simulink model "TWIN"  (R2022a)
settings: Solver=FixedStepAuto  StartTime=0.0  StopTime=20  FixedStep=Ts  RelTol=1000000
values from neighbouring files (symbols this model uses):
  axis_A_init = X(1)    [MOSC_two_axis_machine_key.m]
  axis_B_init = Y(1)    [MOSC_two_axis_machine_key.m]
  c = 0    [MOSC_two_axis_machine_key.m]
  i_offset = 0.01    [MOSC_two_axis_machine_key.m]
  In = 7.2    [MOSC_two_axis_machine_key.m]
  J = (0.013*2)    (= 0.026)    [MOSC_two_axis_machine_key.m]
  k1a = 2    [MOSC_two_axis_machine_key.m]
  k1b = 2    [MOSC_two_axis_machine_key.m]
  k2a = 2    [MOSC_two_axis_machine_key.m]
  k2b = 2    [MOSC_two_axis_machine_key.m]
  k3b = 2    [MOSC_two_axis_machine_key.m]
  k4b = 2    [MOSC_two_axis_machine_key.m]
  k_conv = 350    [MOSC_two_axis_machine_key.m]
  k_meas_i = 10    [MOSC_two_axis_machine_key.m]
  k_meas_w = 5    [MOSC_two_axis_machine_key.m]
  Ki = Kr    (= 0.448835548336)    [MOSC_two_axis_machine_key.m]
  ki_om = K_reg_omega_SO    (= 0.938140461276)    [MOSC_two_axis_machine_key.m]
  Kp = Kr*Tr    (= 0.00161048636688)    [MOSC_two_axis_machine_key.m]
  kp_om = K_reg_omega_SO * T_reg_omega_SO    (= 0.185714285714)    [MOSC_two_axis_machine_key.m]
  kp_pos = 13    [MOSC_two_axis_machine_key.m]
  La = 23e-3    (= 0.023)    [MOSC_two_axis_machine_key.m]
  PSI_E = (Un-Ra*In)/wn    (= 1.36163652923)    [MOSC_two_axis_machine_key.m]
  PSI_M = Tn/In    (= 1.22916666667)    [MOSC_two_axis_machine_key.m]
  Ra = 6.41    [MOSC_two_axis_machine_key.m]
  rand_seed_1 = round(rand*(2^32-1))    [MOSC_two_axis_machine_key.m]
  rand_seed_2 = round(rand*(2^32-1))    [MOSC_two_axis_machine_key.m]
  rand_seed_3 = round(rand*(2^32-1))    [MOSC_two_axis_machine_key.m]
  rand_seed_4 = round(rand*(2^32-1))    [MOSC_two_axis_machine_key.m]
  Tdelay = 2*Ts    (= 0.002)    [MOSC_two_axis_machine_key.m]
  Tn = 8.85    [MOSC_two_axis_machine_key.m]
  Ts = 0.001    [MOSC_two_axis_machine_key.m]
  v_i_a = (In*measurement_noise_level/2)^2    (= 0.001296)    [MOSC_two_axis_machine_key.m]
  w1a = 1*2*pi*frequency_heart    (= 6.28318530718)    [MOSC_two_axis_machine_key.m]
  w1b = 1*2*pi*frequency_heart    (= 6.28318530718)    [MOSC_two_axis_machine_key.m]    (also in MOSC_updates.m = k(1)*1*2*pi*frequency_heart)
  w2a = 3*2*pi*frequency_heart    (= 18.8495559215)    [MOSC_two_axis_machine_key.m]
  w2b = 2*2*pi*frequency_heart    (= 12.5663706144)    [MOSC_two_axis_machine_key.m]    (also in MOSC_updates.m = k(2)*2*2*pi*frequency_heart)
  w3b = 3*2*pi*frequency_heart    (= 18.8495559215)    [MOSC_two_axis_machine_key.m]    (also in MOSC_updates.m = k(3)*3*2*pi*frequency_heart)
  w4b = 4*2*pi*frequency_heart    (= 25.1327412287)    [MOSC_two_axis_machine_key.m]    (also in MOSC_updates.m = k(4)*4*2*pi*frequency_heart)
  w_i_a = (dia_max*system_noise_level/2)^2    (= 2500)    [MOSC_two_axis_machine_key.m]
  w_offset = 0    [MOSC_two_axis_machine_key.m]
  w_omega_m = (domega_max*system_noise_level/2)^2    (= 100)    [MOSC_two_axis_machine_key.m]
  w_u_a = (du_max*system_noise_level/2)^2    (= 25000000)    [MOSC_two_axis_machine_key.m]
  wn = 1640*pi/30    (= 171.740398396)    [MOSC_two_axis_machine_key.m]
  zeta1a = 0.01    [MOSC_two_axis_machine_key.m]
  zeta1b = 0.01    [MOSC_two_axis_machine_key.m]
  zeta2a = 0.01    [MOSC_two_axis_machine_key.m]
  zeta2b = 0.01    [MOSC_two_axis_machine_key.m]
  zeta3b = 0.01    [MOSC_two_axis_machine_key.m]
  zeta4b = 0.01    [MOSC_two_axis_machine_key.m]
libraries: slpidlib x4
settings Model: Creator=nirvana1289  LastModifiedBy=akash
settings SolverCC: ZeroCrossAlgorithm=Adaptive  AlgebraicLoopSolver=TrustRegion
settings DataIOCC: ReturnWorkspaceOutputs=off
settings DebuggingCC: IgnoredZcDiagnostic=none  UnconnectedInputMsg=warning  UnconnectedOutputMsg=warning  UnconnectedLineMsg=warning  SFMachineParentedDataDiag=warning  ArithmeticOperatorsInVariantConditions=warning
settings SFSimCC: SimUseLocalCustomCode=off  CustomCodeUndefinedFunction=UseInterfaceOnly
settings RTWCC: RTWUseLocalCustomCode=off  DLArmComputeVersion=19.05
settings CodeAppCC: StateflowObjectComments=on

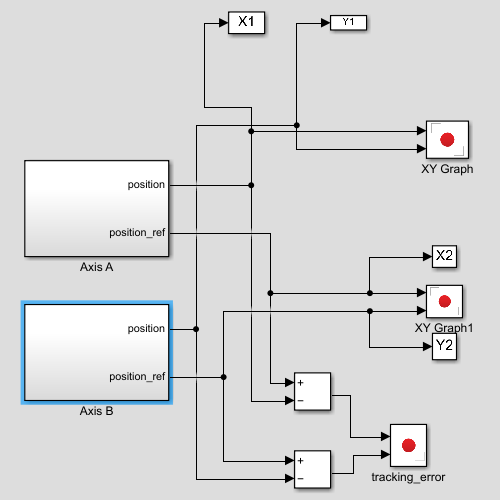
[thumbnail: Simulink's stored preview of the top-level diagram]
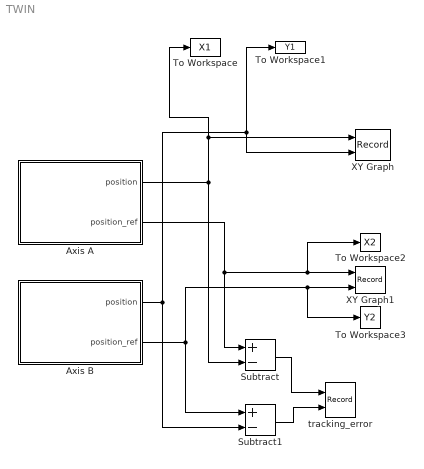
== system TWIN ==
  Axis A : Subsystem
  Axis B : Subsystem
  Subtract : Sum  Inputs=+-
  Subtract1 : Sum  Inputs=+-
  To Workspace : ToWorkspace  VariableName=X1  SampleTime=-1
      settings: Save2DSignal=2-D array (concatenate along first dimension)
  To Workspace1 : ToWorkspace  VariableName=Y1  SampleTime=-1
      settings: Save2DSignal=2-D array (concatenate along first dimension)
  To Workspace2 : ToWorkspace  VariableName=X2  SampleTime=-1
      settings: Save2DSignal=2-D array (concatenate along first dimension)
  To Workspace3 : ToWorkspace  VariableName=Y2  SampleTime=-1
      settings: Save2DSignal=2-D array (concatenate along first dimension)
  XY Graph : Record  FileSettingsInternal="{\"entries\":[{\"content\":{\"excelSettings\":{\"content\":{},\"type\":\"Streamout.ExcelSettings\"}},\"type\":\"Streamout.FileSettingStorage\",\"uuid\":\"5dd5c6a3-9558-46e3-9c57-18c47edfeb62\"}],\"packageUris\":[\"http://schema.mathworks.com/mf0/streamout_blocks/R2020a\"],\"version\":\"1.0\"}"  Layout=[1 1]  SignalsInternal="{\"entries\":[{\"content\":{\"signals\":[{\"content\":{\"blockPath\":[\"TWIN/XY Graph\"],\"channel\":[],\"dimensions\":[1],\"domain\":\"TWIN/XY Graph\",\"lineColor\":\"#a2142f\",\"plots\":[1],\"port\":1,\"sid\":[\"\"],\"signalID\":483759,\"signalName\":\"Axis A:1\"},\"type\":\"RecordBlkView.Signal\",\"uuid\":\"e5131e20-f6b1-48ad-bb87-b3fb0198be33\"},{\"content\":{\"blockPath\":[\"TWIN/XY Graph\"],\"channel\":[],\"dimensions\":[1],\"domain\":\"TWIN/XY Graph\",\"lineColor\":\"#139fff\",\"plots\":[1],\"port\":2,\"sid\":[\"\"],\"signalID\":483763,\"signalName\":\"Axis B:1\"},\"type\":\"RecordBlkView.Signal\",\"uuid\":\"a231155c-1ff8-46a4-b816-94ab751d59c2\"}]},\"type\":\"RecordBlkView.InputSignals\",\"uuid\":\"a1552bf6-88ac-4365-aa89-aa31ab89a906\"}],\"packageUris\":[\"http://schema.mathworks.com/mf0/streamout_blocks/R2020a\"],\"version\":\"1.0\"}"  VisualizationBindings="{\"xyplotplugin\":{\"info\":[{\"series\":[{\"bindingParametersList\":[{\"parameter\":\"X-Axis\",\"signalID\":483759,\"signalName\":\"Axis A:1\"},{\"parameter\":\"Y-Axis\",\"signalID\":483763,\"signalName\":\"Axis B:1\"}],\"seriesID\":45665}],\"subplotID\":1}]}}"  CompatibilityTag=XY
  XY Graph1 : Record  FileSettingsInternal="{\"entries\":[{\"content\":{\"excelSettings\":{\"content\":{},\"type\":\"Streamout.ExcelSettings\"}},\"type\":\"Streamout.FileSettingStorage\",\"uuid\":\"d2fb6019-1089-4865-91d9-d366b06b0246\"}],\"packageUris\":[\"http://schema.mathworks.com/mf0/streamout_blocks/R2020a\"],\"version\":\"1.0\"}"  Layout=[1 1]  SignalsInternal="{\"entries\":[{\"content\":{\"signals\":[{\"content\":{\"blockPath\":[\"TWIN/XY Graph1\"],\"channel\":[],\"dimensions\":[1],\"domain\":\"TWIN/XY Graph1\",\"lineColor\":\"#ff6929\",\"plots\":[],\"port\":1,\"sid\":[\"\"],\"signalID\":483767,\"signalName\":\"Axis A:2\"},\"type\":\"RecordBlkView.Signal\",\"uuid\":\"f7357322-d349-4bee-9fb2-232c0e5c727e\"},{\"content\":{\"blockPath\":[\"TWIN/XY Graph1\"],\"channel\":[],\"dimensions\":[1],\"domain\":\"TWIN/XY Graph1\",\"lineColor\":\"#b746ff\",\"plots\":[],\"port\":2,\"sid\":[\"\"],\"signalID\":483771,\"signalName\":\"Axis B:2\"},\"type\":\"RecordBlkView.Signal\",\"uuid\":\"1ed46889-5323-47ea-b6ba-a8126608ec68\"}]},\"type\":\"RecordBlkView.InputSignals\",\"uuid\":\"2741a743-7749-4c48-8803-007fd9de5a09\"}],\"packageUris\":[\"http://schema.mathworks.com/mf0/streamout_blocks/R2020a\"],\"version\":\"1.0\"}"  VisualizationBindings="{\"xyplotplugin\":{\"info\":[{\"series\":[],\"subplotID\":1}]}}"  CompatibilityTag=XY
  tracking_error : Record  FileSettingsInternal="{\"entries\":[{\"content\":{\"excelSettings\":{\"content\":{},\"type\":\"Streamout.ExcelSettings\"}},\"type\":\"Streamout.FileSettingStorage\",\"uuid\":\"68a8b464-3159-494c-9b13-e187b7557057\"}],\"packageUris\":[\"http://schema.mathworks.com/mf0/streamout_blocks/R2020a\"],\"version\":\"1.0\"}"  Layout=[1 1]  SignalsInternal="{\"entries\":[{\"content\":{\"signals\":[{\"content\":{\"blockPath\":[\"TWIN/tracking_error\"],\"channel\":[],\"dimensions\":[1],\"domain\":\"TWIN/tracking_error\",\"lineColor\":\"#0072bd\",\"plots\":[],\"port\":1,\"sid\":[\"\"],\"signalID\":483791,\"signalName\":\"Subtract\"},\"type\":\"RecordBlkView.Signal\",\"uuid\":\"10eded9b-e3ea-40dd-a408-67c9f9bb2562\"},{\"content\":{\"blockPath\":[\"TWIN/tracking_error\"],\"channel\":[],\"dimensions\":[1],\"domain\":\"TWIN/tracking_error\",\"lineColor\":\"#d95319\",\"plots\":[],\"port\":2,\"sid\":[\"\"],\"signalID\":483795,\"signalName\":\"Subtract1\"},\"type\":\"RecordBlkView.Signal\",\"uuid\":\"27c12579-6568-4ff9-89bb-dc84c731a73d\"}]},\"type\":\"RecordBlkView.InputSignals\",\"uuid\":\"269cb1b5-4398-46da-8bba-8f15a29c1fed\"}],\"packageUris\":[\"http://schema.mathworks.com/mf0/streamout_blocks/R2020a\"],\"version\":\"1.0\"}"  VisualizationBindings="{\"xyplotplugin\":{\"info\":[{\"series\":[],\"subplotID\":1}]}}"  CompatibilityTag=XY  st=-1
  wires:
  Axis B/2(position_ref) -> To Workspace3/1, XY Graph1/2, Subtract1/1
  Subtract1/1 -> tracking_error/2
  Axis B/1(position) -> XY Graph/2, To Workspace1/1, Subtract1/2
  Subtract/1 -> tracking_error/1
  Axis A/1(position) -> To Workspace/1, XY Graph/1, Subtract/2
  Axis A/2(position_ref) -> Subtract/1, To Workspace2/1, XY Graph1/1

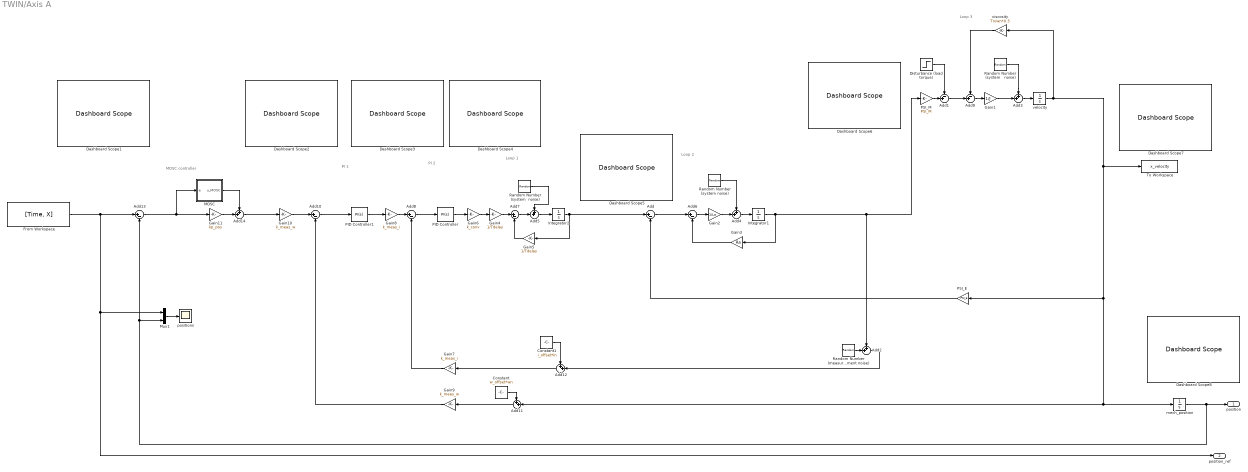
== system TWIN/Axis A ==
  note: Loop 3
  note: Loop 2
  note: Loop 1
  note: PI 2
  note: PI 1
  note: MOSC controller
  Add{,6..8,10,13} (6 alike) : Sum  Inputs=|+-
  Add1 : Sum  Inputs=-+|
  Add{2..5,11..12,14} (7 alike) : Sum  Inputs=++|
  Add9 : Sum  Inputs=-+|
  Constant : Constant  Value=w_offset*wn
  Constant1 : Constant  Value=i_offset*In
  Dashboard Scope{1..8} (8 alike) : DashboardScope
  Disturbance (load torque) : Step  Time=0  After=0  SampleTime=0
  From Workspace : FromWorkspace  VariableName=[Time, X]  OutputAfterFinalValue=Setting to zero
  Gain1 : Gain  Gain=1/J
  Gain10 : Gain  Gain=k_meas_w
  Gain11 : Gain  Gain=kp_pos
  Gain2 : Gain  Gain=1/La
  Gain3 : Gain  Gain=Ra
  Gain4 : Gain  Gain=1/Tdelay
  Gain5 : Gain  Gain=1/Tdelay
  Gain6 : Gain  Gain=k_conv
  Gain7 : Gain  Gain=k_meas_i
  Gain8 : Gain  Gain=k_meas_i
  Gain9 : Gain  Gain=k_meas_w
  Integrator1 : Integrator
  Integrator2 : Integrator
  MOSC : Subsystem
  Mux1 : Mux  Inputs=2
  PID Controller : slpidlib/PID Controller  Controller=PI  Form=Parallel  TimeDomain=Continuous-time  UseExternalTs=off  SampleTime=-1  IntegratorMethod=Forward Euler  FilterMethod=Forward Euler  ControllerParametersSource=internal  P=Kp  I=Ki  UseKiTs=off  D=0  N=100  UseFilter=on  TunerSelectOption=Transfer Function Based (PID Tuner App)  InitialConditionSource=internal  InitialConditionForIntegrator=0  InitialConditionForFilter=0  DifferentiatorICPrevScaledInput=0  ExternalReset=none  TrackingMode=off  Kt=1  LimitOutput=on  SatLimitsSource=internal  UpperSaturationLimit=1  LowerSaturationLimit=-1  LinearizeAsGain=on  AntiWindupMode=clamping  Kb=1  POutMin=[]  POutMax=[]  IOutMin=[]  IOutMax=[]  DOutMin=[]  DOutMax=[]  NOutMin=[]  NOutMax=[]  SumOutMin=[]  SumOutMax=[]  SaturationOutMin=[]  SaturationOutMax=[]  PParamMin=[]  PParamMax=[]  IParamMin=[]  IParamMax=[]  DParamMin=[]  DParamMax=[]  NParamMin=[]  NParamMax=[]  KbParamMin=[]  KbParamMax=[]  KtParamMin=[]  KtParamMax=[]  KbOutMin=[]  KbOutMax=[]  KtOutMin=[]  KtOutMax=[]  IntegratorOutMin=[]  IntegratorOutMax=[]  FilterOutMin=[]  FilterOutMax=[]  SumI1OutMin=[]  SumI1OutMax=[]  SumI2OutMin=[]  SumI2OutMax=[]  SumI3OutMin=[]  SumI3OutMax=[]  SumI4OutMin=[]  SumI4OutMax=[]  SumDOutMin=[]  SumDOutMax=[]  DifferentiatorOutMin=[]  DifferentiatorOutMax=[]  FilterDiffOutCoefMin=[]  FilterDiffOutCoefMax=[]  ReciprocalOutMin=[]  ReciprocalOutMax=[]  SumDenOutMin=[]  SumDenOutMax=[]  SumNumOutMin=[]  SumNumOutMax=[]  DivideOutMin=[]  DivideOutMax=[]  UdiffTsProdOutMin=[]  UdiffTsProdOutMax=[]  NTsProdOutMin=[]  NTsProdOutMax=[]  UintegralTsProdOutMin=[]  UintegralTsProdOutMax=[]  UngainTsProdOutMin=[]  UngainTsProdOutMax=[]  IntegratorContinuousStateAttributes=''  IntegratorStateMustResolveToSignalObject=off  IntegratorRTWStateStorageClass=Auto  FilterContinuousStateAttributes=''  FilterStateMustResolveToSignalObject=off  FilterRTWStateStorageClass=Auto  ParallelPVariant=InternalParameters  IdealPVariant=Disabled  IVariant=InternalParameters  DVariant=Disabled  IntegratorVariant=Continuous  SatVariant=Enabled  AWVariant=ContClampingParallel  PCopyVariant=Disabled  TRVariant=Disabled  FdbkBlocksVariant=Forward  IdealPFdbkVariant=Disabled  SatFdbkVariant=Disabled  DerivativeFilterVariant=Disabled  NVariant=Disabled  NCopyVariant=Disabled_SignalSpec  FilterICVariant=Disabled  IntegratorICVariant=InternalICs  ExternalResetVariant=Disabled  TRSumVariant=Passthrough  SumFdbkVariant=Disabled  SumVariant=Sum_PI  TsampFilterVariant=InternalTs  TsampNgainVariant=Passthrough  TsampIntegralVariant=Passthrough  ExternalSaturationOutDataTypeStr=Inherit: Same as second input  aMode=0
  PID Controller1 : slpidlib/PID Controller  Controller=PI  Form=Parallel  TimeDomain=Continuous-time  UseExternalTs=off  SampleTime=-1  IntegratorMethod=Forward Euler  FilterMethod=Forward Euler  ControllerParametersSource=internal  P=kp_om  I=ki_om  UseKiTs=off  D=0  N=100  UseFilter=on  TunerSelectOption=Transfer Function Based (PID Tuner App)  InitialConditionSource=internal  InitialConditionForIntegrator=0  InitialConditionForFilter=0  DifferentiatorICPrevScaledInput=0  ExternalReset=none  TrackingMode=off  Kt=1  LimitOutput=on  SatLimitsSource=internal  UpperSaturationLimit=In  LowerSaturationLimit=-In  LinearizeAsGain=on  AntiWindupMode=clamping  Kb=500  POutMin=[]  POutMax=[]  IOutMin=[]  IOutMax=[]  DOutMin=[]  DOutMax=[]  NOutMin=[]  NOutMax=[]  SumOutMin=[]  SumOutMax=[]  SaturationOutMin=[]  SaturationOutMax=[]  PParamMin=[]  PParamMax=[]  IParamMin=[]  IParamMax=[]  DParamMin=[]  DParamMax=[]  NParamMin=[]  NParamMax=[]  KbParamMin=[]  KbParamMax=[]  KtParamMin=[]  KtParamMax=[]  KbOutMin=[]  KbOutMax=[]  KtOutMin=[]  KtOutMax=[]  IntegratorOutMin=[]  IntegratorOutMax=[]  FilterOutMin=[]  FilterOutMax=[]  SumI1OutMin=[]  SumI1OutMax=[]  SumI2OutMin=[]  SumI2OutMax=[]  SumI3OutMin=[]  SumI3OutMax=[]  SumI4OutMin=[]  SumI4OutMax=[]  SumDOutMin=[]  SumDOutMax=[]  DifferentiatorOutMin=[]  DifferentiatorOutMax=[]  FilterDiffOutCoefMin=[]  FilterDiffOutCoefMax=[]  ReciprocalOutMin=[]  ReciprocalOutMax=[]  SumDenOutMin=[]  SumDenOutMax=[]  SumNumOutMin=[]  SumNumOutMax=[]  DivideOutMin=[]  DivideOutMax=[]  UdiffTsProdOutMin=[]  UdiffTsProdOutMax=[]  NTsProdOutMin=[]  NTsProdOutMax=[]  UintegralTsProdOutMin=[]  UintegralTsProdOutMax=[]  UngainTsProdOutMin=[]  UngainTsProdOutMax=[]  IntegratorContinuousStateAttributes=''  IntegratorStateMustResolveToSignalObject=off  IntegratorRTWStateStorageClass=Auto  FilterContinuousStateAttributes=''  FilterStateMustResolveToSignalObject=off  FilterRTWStateStorageClass=Auto  ParallelPVariant=InternalParameters  IdealPVariant=Disabled  IVariant=InternalParameters  DVariant=Disabled  IntegratorVariant=Continuous  SatVariant=Enabled  AWVariant=ContClampingParallel  PCopyVariant=Disabled  TRVariant=Disabled  FdbkBlocksVariant=Forward  IdealPFdbkVariant=Disabled  SatFdbkVariant=Disabled  DerivativeFilterVariant=Disabled  NVariant=Disabled  NCopyVariant=Disabled_SignalSpec  FilterICVariant=Disabled  IntegratorICVariant=InternalICs  ExternalResetVariant=Disabled  TRSumVariant=Passthrough  SumFdbkVariant=Disabled  SumVariant=Sum_PI  TsampFilterVariant=InternalTs  TsampNgainVariant=Passthrough  TsampIntegralVariant=Passthrough  ExternalSaturationOutDataTypeStr=Inherit: Same as second input  aMode=0
  PSI_E : Gain  Gain=PSI_E
  PSI_M : Gain  Gain=PSI_M
  Random Number (measurement noise) : RandomNumber  Variance=v_i_a*c  Seed=rand_seed_4  SampleTime=Ts
  Random Number (system   noise) : RandomNumber  Variance=w_omega_m*c  Seed=rand_seed_3  SampleTime=Ts
  Random Number (system  noise) : RandomNumber  Variance=w_u_a*c  Seed=rand_seed_1  SampleTime=Ts
  Random Number (system noise) : RandomNumber  Variance=w_i_a*c  Seed=rand_seed_2  SampleTime=Ts
  To Workspace : ToWorkspace  VariableName=x_velocity  SaveFormat=Timeseries  SampleTime=-1
  mech_position : Integrator  InitialCondition=axis_A_init
  positions : Scope
  velocity : Integrator
  viscosity : Gain  Gain=Tn/wn*0.3
  position : Outport
  position_ref : Outport  Port=2
  wires:
  Random Number (system  noise)/1 -> Add5/1
  Gain5/1 -> Add7/2
  Add3/1 -> velocity/1
  Add/1 -> Add6/1
  Gain1/1 -> Add3/2
  Gain3/1 -> Add6/2
  Random Number (measurement noise)/1 -> Add2/2
  PSI_M/1 -> Add1/2
  Random Number (system   noise)/1 -> Add3/1
  Random Number (system noise)/1 -> Add4/1
  Add6/1 -> Gain2/1
  Gain4/1 -> Add7/1
  velocity/1 -> PSI_E/1, Add11/2, mech_position/1, To Workspace/1, viscosity/1
  PSI_E/1 -> Add/2
  Add5/1 -> Integrator2/1
  Add4/1 -> Integrator1/1
  Integrator2/1 -> Add/1, Gain5/1
  Add7/1 -> Add5/2
  PID Controller/1 -> Gain6/1
  Add1/1 -> Add9/2
  viscosity/1 -> Add9/1
  Gain11/1 -> Add14/2
  Gain7/1 -> Add8/2
  Gain2/1 -> Add4/2
  Gain6/1 -> Gain4/1
  Add9/1 -> Gain1/1
  Add2/1 -> Add12/2
  Disturbance (load torque)/1 -> Add1/1
  Integrator1/1 -> Gain3/1, PSI_M/1, Add2/1
  Add10/1 -> PID Controller1/1
  Constant1/1 -> Add12/1
  Gain10/1 -> Add10/1
  Mux1/1 -> positions/1
  PID Controller1/1 -> Gain8/1
  Add8/1 -> PID Controller/1
  Gain8/1 -> Add8/1
  Add12/1 -> Gain7/1
  Add13/1 -> Gain11/1, MOSC/1(e)
  From Workspace/1 -> Add13/1, position_ref/1, Mux1/1
  Add11/1 -> Gain9/1
  Gain9/1 -> Add10/2
  mech_position/1 -> position/1, Add13/2, Mux1/2
  Add14/1 -> Gain10/1
  Constant/1 -> Add11/1
  MOSC/1(u_MOSC) -> Add14/1

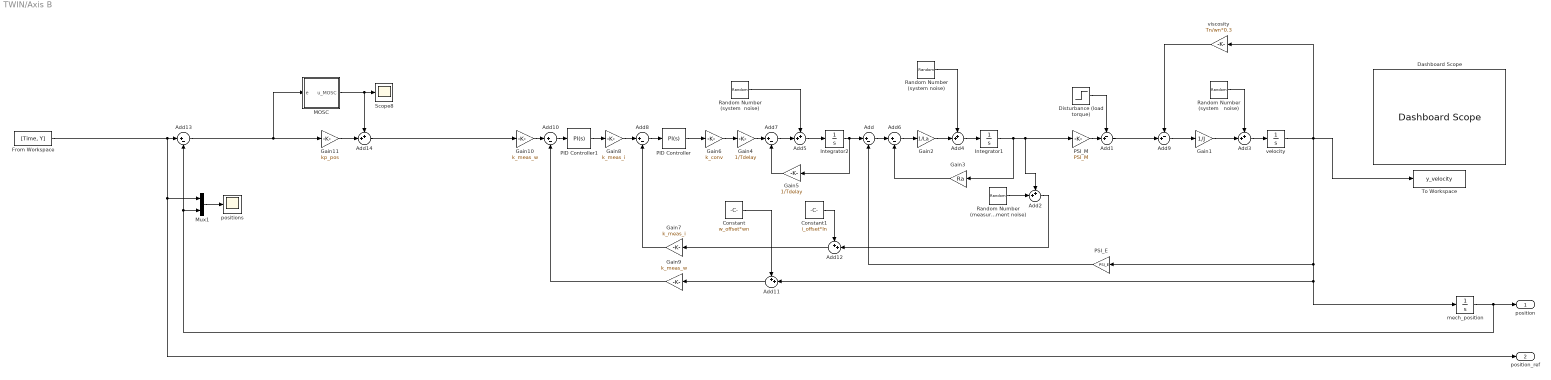
== system TWIN/Axis B ==
  Add{,6..8,10,13} (6 alike) : Sum  Inputs=|+-
  Add1 : Sum  Inputs=-+|
  Add{2..5,11..12,14} (7 alike) : Sum  Inputs=++|
  Add9 : Sum  Inputs=-+|
  Constant : Constant  Value=w_offset*wn
  Constant1 : Constant  Value=i_offset*In
  Dashboard Scope : DashboardScope
  Disturbance (load torque) : Step  Time=0  After=0  SampleTime=0
  From Workspace : FromWorkspace  VariableName=[Time, Y]  OutputAfterFinalValue=Setting to zero
  Gain1 : Gain  Gain=1/J
  Gain10 : Gain  Gain=k_meas_w
  Gain11 : Gain  Gain=kp_pos
  Gain2 : Gain  Gain=1/La
  Gain3 : Gain  Gain=Ra
  Gain4 : Gain  Gain=1/Tdelay
  Gain5 : Gain  Gain=1/Tdelay
  Gain6 : Gain  Gain=k_conv
  Gain7 : Gain  Gain=k_meas_i
  Gain8 : Gain  Gain=k_meas_i
  Gain9 : Gain  Gain=k_meas_w
  Integrator1 : Integrator
  Integrator2 : Integrator
  MOSC : Subsystem
  Mux1 : Mux  Inputs=2
  PID Controller : slpidlib/PID Controller  Controller=PI  Form=Parallel  TimeDomain=Continuous-time  UseExternalTs=off  SampleTime=-1  IntegratorMethod=Forward Euler  FilterMethod=Forward Euler  ControllerParametersSource=internal  P=Kp  I=Ki  UseKiTs=off  D=0  N=100  UseFilter=on  TunerSelectOption=Transfer Function Based (PID Tuner App)  InitialConditionSource=internal  InitialConditionForIntegrator=0  InitialConditionForFilter=0  DifferentiatorICPrevScaledInput=0  ExternalReset=none  TrackingMode=off  Kt=1  LimitOutput=on  SatLimitsSource=internal  UpperSaturationLimit=1  LowerSaturationLimit=-1  LinearizeAsGain=on  AntiWindupMode=clamping  Kb=1  POutMin=[]  POutMax=[]  IOutMin=[]  IOutMax=[]  DOutMin=[]  DOutMax=[]  NOutMin=[]  NOutMax=[]  SumOutMin=[]  SumOutMax=[]  SaturationOutMin=[]  SaturationOutMax=[]  PParamMin=[]  PParamMax=[]  IParamMin=[]  IParamMax=[]  DParamMin=[]  DParamMax=[]  NParamMin=[]  NParamMax=[]  KbParamMin=[]  KbParamMax=[]  KtParamMin=[]  KtParamMax=[]  KbOutMin=[]  KbOutMax=[]  KtOutMin=[]  KtOutMax=[]  IntegratorOutMin=[]  IntegratorOutMax=[]  FilterOutMin=[]  FilterOutMax=[]  SumI1OutMin=[]  SumI1OutMax=[]  SumI2OutMin=[]  SumI2OutMax=[]  SumI3OutMin=[]  SumI3OutMax=[]  SumI4OutMin=[]  SumI4OutMax=[]  SumDOutMin=[]  SumDOutMax=[]  DifferentiatorOutMin=[]  DifferentiatorOutMax=[]  FilterDiffOutCoefMin=[]  FilterDiffOutCoefMax=[]  ReciprocalOutMin=[]  ReciprocalOutMax=[]  SumDenOutMin=[]  SumDenOutMax=[]  SumNumOutMin=[]  SumNumOutMax=[]  DivideOutMin=[]  DivideOutMax=[]  UdiffTsProdOutMin=[]  UdiffTsProdOutMax=[]  NTsProdOutMin=[]  NTsProdOutMax=[]  UintegralTsProdOutMin=[]  UintegralTsProdOutMax=[]  UngainTsProdOutMin=[]  UngainTsProdOutMax=[]  IntegratorContinuousStateAttributes=''  IntegratorStateMustResolveToSignalObject=off  IntegratorRTWStateStorageClass=Auto  FilterContinuousStateAttributes=''  FilterStateMustResolveToSignalObject=off  FilterRTWStateStorageClass=Auto  ParallelPVariant=InternalParameters  IdealPVariant=Disabled  IVariant=InternalParameters  DVariant=Disabled  IntegratorVariant=Continuous  SatVariant=Enabled  AWVariant=ContClampingParallel  PCopyVariant=Disabled  TRVariant=Disabled  FdbkBlocksVariant=Forward  IdealPFdbkVariant=Disabled  SatFdbkVariant=Disabled  DerivativeFilterVariant=Disabled  NVariant=Disabled  NCopyVariant=Disabled_SignalSpec  FilterICVariant=Disabled  IntegratorICVariant=InternalICs  ExternalResetVariant=Disabled  TRSumVariant=Passthrough  SumFdbkVariant=Disabled  SumVariant=Sum_PI  TsampFilterVariant=InternalTs  TsampNgainVariant=Passthrough  TsampIntegralVariant=Passthrough  ExternalSaturationOutDataTypeStr=Inherit: Same as second input  aMode=0
  PID Controller1 : slpidlib/PID Controller  Controller=PI  Form=Parallel  TimeDomain=Continuous-time  UseExternalTs=off  SampleTime=-1  IntegratorMethod=Forward Euler  FilterMethod=Forward Euler  ControllerParametersSource=internal  P=kp_om  I=ki_om  UseKiTs=off  D=0  N=100  UseFilter=on  TunerSelectOption=Transfer Function Based (PID Tuner App)  InitialConditionSource=internal  InitialConditionForIntegrator=0  InitialConditionForFilter=0  DifferentiatorICPrevScaledInput=0  ExternalReset=none  TrackingMode=off  Kt=1  LimitOutput=on  SatLimitsSource=internal  UpperSaturationLimit=In  LowerSaturationLimit=-In  LinearizeAsGain=on  AntiWindupMode=clamping  Kb=500  POutMin=[]  POutMax=[]  IOutMin=[]  IOutMax=[]  DOutMin=[]  DOutMax=[]  NOutMin=[]  NOutMax=[]  SumOutMin=[]  SumOutMax=[]  SaturationOutMin=[]  SaturationOutMax=[]  PParamMin=[]  PParamMax=[]  IParamMin=[]  IParamMax=[]  DParamMin=[]  DParamMax=[]  NParamMin=[]  NParamMax=[]  KbParamMin=[]  KbParamMax=[]  KtParamMin=[]  KtParamMax=[]  KbOutMin=[]  KbOutMax=[]  KtOutMin=[]  KtOutMax=[]  IntegratorOutMin=[]  IntegratorOutMax=[]  FilterOutMin=[]  FilterOutMax=[]  SumI1OutMin=[]  SumI1OutMax=[]  SumI2OutMin=[]  SumI2OutMax=[]  SumI3OutMin=[]  SumI3OutMax=[]  SumI4OutMin=[]  SumI4OutMax=[]  SumDOutMin=[]  SumDOutMax=[]  DifferentiatorOutMin=[]  DifferentiatorOutMax=[]  FilterDiffOutCoefMin=[]  FilterDiffOutCoefMax=[]  ReciprocalOutMin=[]  ReciprocalOutMax=[]  SumDenOutMin=[]  SumDenOutMax=[]  SumNumOutMin=[]  SumNumOutMax=[]  DivideOutMin=[]  DivideOutMax=[]  UdiffTsProdOutMin=[]  UdiffTsProdOutMax=[]  NTsProdOutMin=[]  NTsProdOutMax=[]  UintegralTsProdOutMin=[]  UintegralTsProdOutMax=[]  UngainTsProdOutMin=[]  UngainTsProdOutMax=[]  IntegratorContinuousStateAttributes=''  IntegratorStateMustResolveToSignalObject=off  IntegratorRTWStateStorageClass=Auto  FilterContinuousStateAttributes=''  FilterStateMustResolveToSignalObject=off  FilterRTWStateStorageClass=Auto  ParallelPVariant=InternalParameters  IdealPVariant=Disabled  IVariant=InternalParameters  DVariant=Disabled  IntegratorVariant=Continuous  SatVariant=Enabled  AWVariant=ContClampingParallel  PCopyVariant=Disabled  TRVariant=Disabled  FdbkBlocksVariant=Forward  IdealPFdbkVariant=Disabled  SatFdbkVariant=Disabled  DerivativeFilterVariant=Disabled  NVariant=Disabled  NCopyVariant=Disabled_SignalSpec  FilterICVariant=Disabled  IntegratorICVariant=InternalICs  ExternalResetVariant=Disabled  TRSumVariant=Passthrough  SumFdbkVariant=Disabled  SumVariant=Sum_PI  TsampFilterVariant=InternalTs  TsampNgainVariant=Passthrough  TsampIntegralVariant=Passthrough  ExternalSaturationOutDataTypeStr=Inherit: Same as second input  aMode=0
  PSI_E : Gain  Gain=PSI_E
  PSI_M : Gain  Gain=PSI_M
  Random Number (measurement noise) : RandomNumber  Variance=v_i_a*c  Seed=rand_seed_4  SampleTime=Ts
  Random Number (system   noise) : RandomNumber  Variance=w_omega_m*c  Seed=rand_seed_3  SampleTime=Ts
  Random Number (system  noise) : RandomNumber  Variance=w_u_a*c  Seed=rand_seed_1  SampleTime=Ts
  Random Number (system noise) : RandomNumber  Variance=w_i_a*c  Seed=rand_seed_2  SampleTime=Ts
  Scope8 : Scope
  To Workspace : ToWorkspace  VariableName=y_velocity  SaveFormat=Timeseries  SampleTime=-1
  mech_position : Integrator  InitialCondition=axis_B_init
  positions : Scope
  velocity : Integrator
  viscosity : Gain  Gain=Tn/wn*0.3
  position : Outport
  position_ref : Outport  Port=2
  wires:
  Random Number (system  noise)/1 -> Add5/1
  Gain5/1 -> Add7/2
  Add3/1 -> velocity/1
  Add/1 -> Add6/1
  Gain1/1 -> Add3/2
  Gain3/1 -> Add6/2
  Random Number (measurement noise)/1 -> Add2/2
  PSI_M/1 -> Add1/2
  Random Number (system   noise)/1 -> Add3/1
  Random Number (system noise)/1 -> Add4/1
  Add6/1 -> Gain2/1
  Gain4/1 -> Add7/1
  velocity/1 -> To Workspace/1, mech_position/1, Add11/2, PSI_E/1, viscosity/1
  PSI_E/1 -> Add/2
  Add5/1 -> Integrator2/1
  Add4/1 -> Integrator1/1
  Integrator2/1 -> Add/1, Gain5/1
  Add7/1 -> Add5/2
  PID Controller/1 -> Gain6/1
  Add1/1 -> Add9/2
  viscosity/1 -> Add9/1
  Gain11/1 -> Add14/2
  Gain7/1 -> Add8/2
  Gain2/1 -> Add4/2
  Gain6/1 -> Gain4/1
  Add9/1 -> Gain1/1
  Add2/1 -> Add12/2
  Disturbance (load torque)/1 -> Add1/1
  Integrator1/1 -> Gain3/1, PSI_M/1, Add2/1
  Add10/1 -> PID Controller1/1
  Constant1/1 -> Add12/1
  Gain10/1 -> Add10/1
  Mux1/1 -> positions/1
  PID Controller1/1 -> Gain8/1
  Add8/1 -> PID Controller/1
  Gain8/1 -> Add8/1
  Add12/1 -> Gain7/1
  Add13/1 -> MOSC/1(e), Gain11/1
  From Workspace/1 -> Add13/1, position_ref/1, Mux1/1
  Add11/1 -> Gain9/1
  Gain9/1 -> Add10/2
  mech_position/1 -> Add13/2, Mux1/2, position/1
  Add14/1 -> Gain10/1
  Constant/1 -> Add11/1
  MOSC/1(u_MOSC) -> Scope8/1, Add14/1

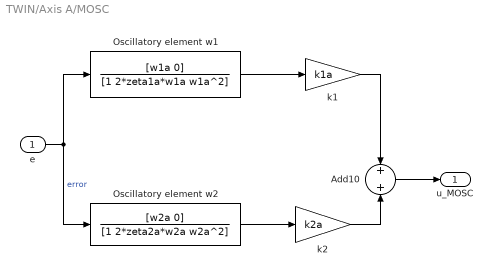
== system TWIN/Axis A/MOSC ==
  e : Inport
  Add10 : Sum
  Oscillatory element w1 : TransferFcn  Numerator=[w1a 0]  Denominator=[1 2*zeta1a*w1a w1a^2]
  Oscillatory element w2 : TransferFcn  Numerator=[w2a 0]  Denominator=[1 2*zeta2a*w2a w2a^2]
  k1 : Gain  Gain=k1a
  k2 : Gain  Gain=k2a
  u_MOSC : Outport
  wires:
  Add10/1 -> u_MOSC/1
  e/1 -> Oscillatory element w2/1, Oscillatory element w1/1  "error"
  Oscillatory element w1/1 -> k1/1
  Oscillatory element w2/1 -> k2/1
  k1/1 -> Add10/1
  k2/1 -> Add10/2

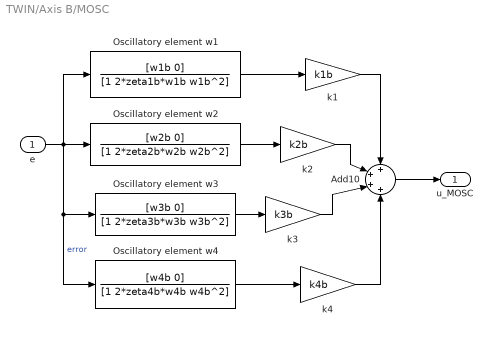
== system TWIN/Axis B/MOSC ==
  e : Inport
  Add10 : Sum  Inputs=++++
  Oscillatory element w1 : TransferFcn  Numerator=[w1b 0]  Denominator=[1 2*zeta1b*w1b w1b^2]
  Oscillatory element w2 : TransferFcn  Numerator=[w2b 0]  Denominator=[1 2*zeta2b*w2b w2b^2]
  Oscillatory element w3 : TransferFcn  Numerator=[w3b 0]  Denominator=[1 2*zeta3b*w3b w3b^2]
  Oscillatory element w4 : TransferFcn  Numerator=[w4b 0]  Denominator=[1 2*zeta4b*w4b w4b^2]
  k1 : Gain  Gain=k1b
  k2 : Gain  Gain=k2b
  k3 : Gain  Gain=k3b
  k4 : Gain  Gain=k4b
  u_MOSC : Outport
  wires:
  Add10/1 -> u_MOSC/1
  e/1 -> Oscillatory element w3/1, Oscillatory element w4/1, Oscillatory element w2/1, Oscillatory element w1/1  "error"
  Oscillatory element w2/1 -> k2/1
  k1/1 -> Add10/1
  Oscillatory element w3/1 -> k3/1
  Oscillatory element w4/1 -> k4/1
  k2/1 -> Add10/2
  k3/1 -> Add10/3
  k4/1 -> Add10/4
  Oscillatory element w1/1 -> k1/1
